simulink model "IEEE_1547_Testing_PHIL"  (R2023b)
settings: Solver=ode4  StartTime=0.0  StopTime=inf  FixedStep=Ts  RelTol=1e-3
PostLoadFcn:
  | init;
InitFcn:
  | init;
undefined symbols (not defined in the file): another_event_name, CURRENT_INPUT_OFFSET_PHA, CURRENT_INPUT_OFFSET_PHB, CURRENT_INPUT_OFFSET_PHC, CURRENT_INPUT_SCALE_PHA, CURRENT_INPUT_SCALE_PHB, CURRENT_INPUT_SCALE_PHC, DiscIntNeverNeededParam, ENABLE_PHA, ENABLE_PHB, ENABLE_PHC, EX, FNOM, FREQUENCY, FREQUENCY_MAX_LIMIT, FREQUENCY_MIN_LIMIT, FRT_CONDITION, FRT_END_TIMING, FRT_START_TIMING, FRT_VALUES, gcbh, magnitude, MODE, my_event_name, Newton, PCRT_CONDITION, PCRT_END_TIMING, PCRT_START_TIMING, PCRT_VALUES, PHASE, PHNOM, Pnom, Raphson, RMS_ENABLE, ROCOF_ENABLE, ROCOF_INIT, ROCOF_VALUE, ROCOM_ENABLE, ROCOM_END_TIME, ROCOM_INIT, ROCOM_START_TIME, ROCOM_VALUE, sps_rtmsupport, Srated, TE0741_4, Ts, TwoSSS_AIO_CPWM, VNOM, VOLT_INPUT_OFFSET_PHA, VOLT_INPUT_OFFSET_PHB, VOLT_INPUT_OFFSET_PHC, VOLT_INPUT_SCALE_PHA, VOLT_INPUT_SCALE_PHB, VOLT_INPUT_SCALE_PHC, VOLT_OUTPUT_SCALE_PHA, VOLT_OUTPUT_SCALE_PHB, VOLT_OUTPUT_SCALE_PHC, VOLTAGE, VOLTAGE_MAX_LIMIT, VOLTAGE_MIN_LIMIT ... (+8)
libraries: simulink x14, rtlab x6, simulink_extras x6, spsFourierLib x6, spsMeanLib x6, rtio_opalrt_common x4, eePowerMeasurement x3, spsPLL3phLib x1, spspowerguiLib x1
(part 2 of 2)

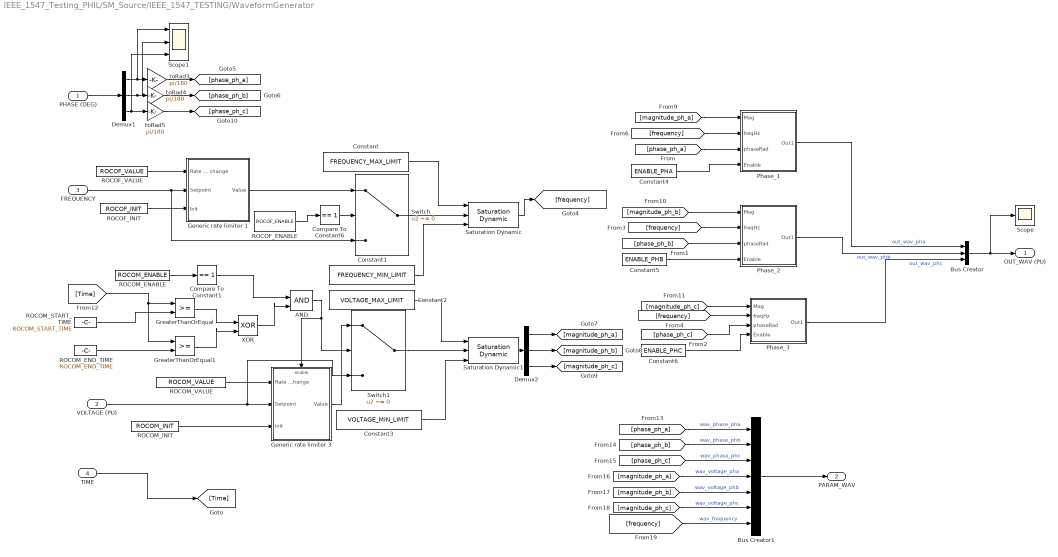
== system IEEE_1547_Testing_PHIL/SM_Source/IEEE_1547_TESTING/WaveformGenerator ==
  PHASE (DEG) : Inport
  VOLTAGE (PU) : Inport  Port=2
  FREQUENCY : Inport  Port=3
  TIME : Inport  Port=4
  AND : Logic  IconShape=distinctive  AllPortsSameDT=off  OutDataTypeStr=boolean
  Bus Creator : BusCreator  Inputs=3
  Bus Creator1 : BusCreator  Inputs=7
  Compare To Constant1 : simulink/Logic and Bit Operations/Compare To Constant  relop===  const=1  OutDataTypeStr=boolean
  Compare To Constant6 : simulink/Logic and Bit Operations/Compare To Constant  relop===  const=1  OutDataTypeStr=boolean
  Constant : Constant  Value=FREQUENCY_MAX_LIMIT
  Constant1 : Constant  Value=FREQUENCY_MIN_LIMIT
  Constant2 : Constant  Value=VOLTAGE_MAX_LIMIT
  Constant3 : Constant  Value=VOLTAGE_MIN_LIMIT
  Constant4 : Constant  Value=ENABLE_PHA
  Constant5 : Constant  Value=ENABLE_PHB
  Constant6 : Constant  Value=ENABLE_PHC
  Demux1 : Demux  Outputs=3
  Demux2 : Demux  Outputs=3
  Generic rate limiter 1 : Subsystem
  Generic rate limiter 3 : Subsystem
  GreaterThanOrEqual : RelationalOperator  OutDataTypeStr=boolean  RndMeth=Simplest  InputSameDT=off
  GreaterThanOrEqual1 : RelationalOperator  OutDataTypeStr=boolean  RndMeth=Simplest  InputSameDT=off
  Phase_1 : Subsystem
  Phase_2 : Subsystem
  Phase_3 : Subsystem
  ROCOF_ENABLE : Constant  Value=ROCOF_ENABLE
  ROCOF_INIT : Constant  Value=ROCOF_INIT
  ROCOF_VALUE : Constant  Value=ROCOF_VALUE
  ROCOM_ENABLE : Constant  Value=ROCOM_ENABLE
  ROCOM_END_TIME : Constant  Value=ROCOM_END_TIME
  ROCOM_INIT : Constant  Value=ROCOM_INIT
  ROCOM_START_TIME : Constant  Value=ROCOM_START_TIME
  ROCOM_VALUE : Constant  Value=ROCOM_VALUE
  Saturation Dynamic : simulink/Discontinuities/Saturation Dynamic  OutMin=[]  OutMax=[]  OutDataTypeStr=Inherit: Same as second input  OutDataType=fixdt(1, 16)  OutScaling=2^-10  DoSatur=off
  Saturation Dynamic1 : simulink/Discontinuities/Saturation Dynamic  OutMin=[]  OutMax=[]  OutDataTypeStr=Inherit: Same as second input  OutDataType=fixdt(1, 16)  OutScaling=2^-10  DoSatur=off
  Scope : Scope
  Scope1 : Scope  NumInputPorts=3
  Switch : Switch  Criteria=u2 ~= 0  SaturateOnIntegerOverflow=off  InputSameDT=off
  Switch1 : Switch  Criteria=u2 ~= 0  SaturateOnIntegerOverflow=off  InputSameDT=off
  XOR : Logic  Operator=XOR  IconShape=distinctive  AllPortsSameDT=off  OutDataTypeStr=boolean
  toRad3 : Gain  Gain=pi/180
  toRad4 : Gain  Gain=pi/180
  toRad5 : Gain  Gain=pi/180
  OUT_WAV (PU) : Outport
  PARAM_WAV : Outport  Port=2
  wires:
  VOLTAGE (PU)/1 -> Switch1/3, Generic rate limiter 3/2("Setpoint ")
  [phase_ph_a] -> Phase_1/3(phaseRad)
  [phase_ph_b] -> Phase_2/3(phaseRad)
  [phase_ph_c] -> Phase_3/3(phaseRad)
  Generic rate limiter 1/1(Value) -> Switch/1
  FREQUENCY/1 -> Switch/3, Generic rate limiter 1/2("Setpoint ")
  ROCOF_VALUE/1 -> Generic rate limiter 1/1(Rate of change)
  ROCOF_INIT/1 -> Generic rate limiter 1/3(Init)
  ROCOF_ENABLE/1 -> Compare To Constant6/1
  Compare To Constant6/1 -> Switch/2
  ROCOM_VALUE/1 -> Generic rate limiter 3/1(Rate of change)
  ROCOM_INIT/1 -> Generic rate limiter 3/3(Init)
  [frequency] -> Phase_1/2(freqHz)
  [frequency] -> Phase_2/2(freqHz)
  Demux2/1 -> [magnitude_ph_a]
  Demux2/2 -> [magnitude_ph_b]
  Demux2/3 -> [magnitude_ph_c]
  [magnitude_ph_a] -> Phase_1/1(Mag)
  [magnitude_ph_b] -> Phase_2/1(Mag)
  [magnitude_ph_c] -> Phase_3/1(Mag)
  [Time] -> GreaterThanOrEqual1/1, GreaterThanOrEqual/1
  ROCOM_START_TIME/1 -> GreaterThanOrEqual/2
  ROCOM_END_TIME/1 -> GreaterThanOrEqual1/2
  GreaterThanOrEqual/1 -> XOR/1
  GreaterThanOrEqual1/1 -> XOR/2
  Switch1/1 -> Saturation Dynamic1/2
  Generic rate limiter 3/1(Value) -> Switch1/1
  AND/1 -> Switch1/2, Generic rate limiter 3/Enable
  XOR/1 -> AND/2
  Compare To Constant1/1 -> AND/1
  ROCOM_ENABLE/1 -> Compare To Constant1/1
  Switch/1 -> Saturation Dynamic/2
  TIME/1 -> [Time]
  Phase_1/1(Out1) -> Bus Creator/1  "out_wav_pha"
  Phase_2/1(Out1) -> Bus Creator/2  "out_wav_phb"
  Phase_3/1(Out1) -> Bus Creator/3  "out_wav_phc"
  Bus Creator/1 -> Scope/1, OUT_WAV (PU)/1
  [phase_ph_a] -> Bus Creator1/1  "wav_phase_pha"
  [phase_ph_b] -> Bus Creator1/2  "wav_phase_phb"
  [phase_ph_c] -> Bus Creator1/3  "wav_phase_phc"
  [magnitude_ph_a] -> Bus Creator1/4  "wav_voltage_pha"
  [magnitude_ph_b] -> Bus Creator1/5  "wav_voltage_phb"
  [magnitude_ph_c] -> Bus Creator1/6  "wav_voltage_phc"
  [frequency] -> Bus Creator1/7  "wav_frequency"
  Bus Creator1/1 -> PARAM_WAV/1
  Saturation Dynamic/1 -> [frequency]
  Saturation Dynamic1/1 -> Demux2/1
  Constant/1 -> Saturation Dynamic/1
  Constant1/1 -> Saturation Dynamic/3
  Constant2/1 -> Saturation Dynamic1/1
  Constant3/1 -> Saturation Dynamic1/3
  Constant4/1 -> Phase_1/4(Enable)
  Constant5/1 -> Phase_2/4(Enable)
  [frequency] -> Phase_3/2(freqHz)
  Constant6/1 -> Phase_3/4(Enable)
  toRad4/1 -> [phase_ph_b]
  toRad3/1 -> [phase_ph_a]
  toRad5/1 -> [phase_ph_c]
  Demux1/2 -> Scope1/2, toRad4/1
  PHASE (DEG)/1 -> Demux1/1
  Demux1/3 -> toRad5/1, Scope1/3
  Demux1/1 -> Scope1/1, toRad3/1

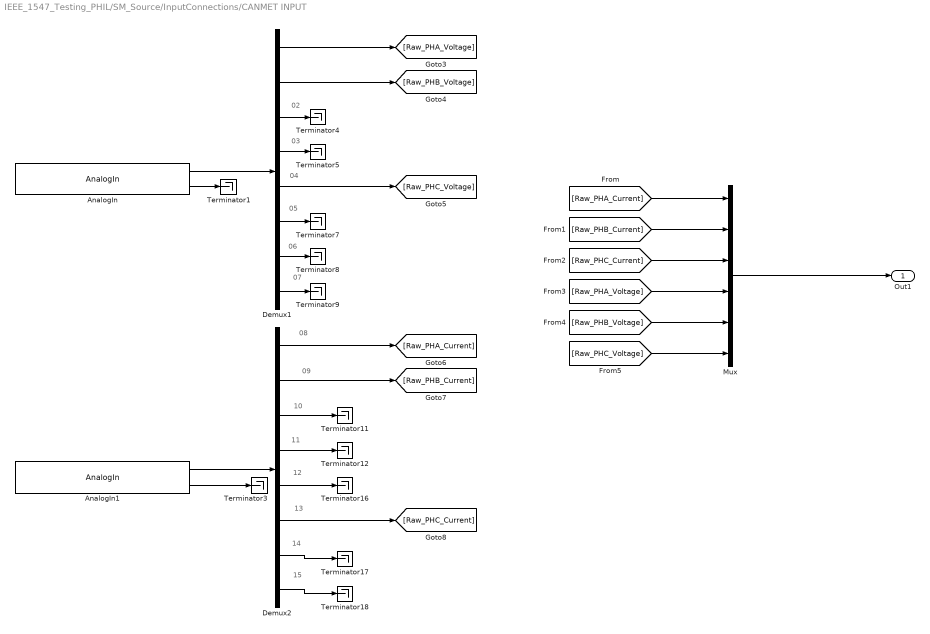
== system IEEE_1547_Testing_PHIL/SM_Source/InputConnections/CANMET INPUT ==
  note: 10
  note: 08
  note: 03
  note: 04
  note: 15
  note: 12
  note: 09
  note: 06
  note: 11
  note: 07
  note: 05
  note: 02
  note: 13
  note: 14
  AnalogIn : rtio_opalrt_common/AnalogIn  CtrlName='OpCtrl'  portNb=7  FcnNos=Slot 6 Module A Subsection 1  size=16  maxcount=8  count=8  numchan=8  sampleTime=0
      settings: AttributesFormatString=%<CtrlName>  SourceProductName=RT-LAB I/O
  AnalogIn1 : rtio_opalrt_common/AnalogIn  CtrlName='OpCtrl'  portNb=8  FcnNos=Slot 6 Module A Subsection 2  size=16  maxcount=8  count=8  numchan=8  sampleTime=0
      settings: AttributesFormatString=%<CtrlName>  SourceProductName=RT-LAB I/O
  Demux1 : Demux  Outputs=8
  Demux2 : Demux  Outputs=8
  Mux : Mux  Inputs=6
  Terminator{1,3..5,7..9,11..12,16..18} (12 alike) : Terminator
  Out1 : Outport  VectorParamsAs1DForOutWhenUnconnected=off
  wires:
  AnalogIn/2 -> Terminator1/1
  AnalogIn1/2 -> Terminator3/1
  AnalogIn/1 -> Demux1/1
  Demux1/4 -> Terminator5/1
  Demux1/7 -> Terminator8/1
  Demux1/6 -> Terminator7/1
  Demux1/8 -> Terminator9/1
  Demux1/3 -> Terminator4/1
  AnalogIn1/1 -> Demux2/1
  Demux2/4 -> Terminator12/1
  Demux2/3 -> Terminator11/1
  Demux2/7 -> Terminator17/1
  Demux2/8 -> Terminator18/1
  Demux2/1 -> [Raw_PHA_Current]
  Demux2/2 -> [Raw_PHB_Current]
  Demux1/5 -> [Raw_PHC_Voltage]
  Demux1/1 -> [Raw_PHA_Voltage]
  Demux1/2 -> [Raw_PHB_Voltage]
  [Raw_PHC_Current] -> Mux/3
  [Raw_PHB_Current] -> Mux/2
  [Raw_PHA_Current] -> Mux/1
  [Raw_PHA_Voltage] -> Mux/4
  [Raw_PHB_Voltage] -> Mux/5
  [Raw_PHC_Voltage] -> Mux/6
  Mux/1 -> Out1/1
  Demux2/5 -> Terminator16/1
  Demux2/6 -> [Raw_PHC_Current]

== system IEEE_1547_Testing_PHIL/SM_Source/IEEE_1547_TESTING/DataAcquisitionSystem/Subsystem ==
  In1 : Inport
  Enable : EnablePort
  FILE_LIMIT : Gain
  FILE_STATUS : Gain
  OpWriteFile : rtlab/DataLogging/OpWriteFile  Static_File=on  varname=Data  Filename=Data.mat  rtpath='./'  nrtpath='.\'  Acq_Group=27  file_size=2.6112e07  write_offline=off  Sim_Mode=off  Nb_Samples=1000  Buffer_size=136000
      settings: SourceProductName=RT-LAB  Decimation=25
  Terminator : Terminator
  Terminator1 : Terminator
  wires:
  OpWriteFile/1 -> FILE_LIMIT/1
  FILE_LIMIT/1 -> Terminator/1
  OpWriteFile/2 -> FILE_STATUS/1
  FILE_STATUS/1 -> Terminator1/1
  In1/1 -> OpWriteFile/1

== system IEEE_1547_Testing_PHIL/SM_Source/IEEE_1547_TESTING/DataAcquisitionSystem/Subsystem1 ==
  In1 : Inport
  Enable : EnablePort
  FILE_LIMIT : Gain
  FILE_STATUS : Gain
  OpWriteFile : rtlab/DataLogging/OpWriteFile  Static_File=on  varname=Data  Filename=WAV.mat  rtpath='./'  nrtpath='.\'  Acq_Group=28  file_size=3e+8  write_offline=off  Sim_Mode=off  Nb_Samples=1000  Buffer_size=200000
      settings: SourceProductName=RT-LAB  Decimation=4
  Terminator : Terminator
  Terminator1 : Terminator
  wires:
  In1/1 -> OpWriteFile/1
  FILE_STATUS/1 -> Terminator1/1
  OpWriteFile/2 -> FILE_STATUS/1
  FILE_LIMIT/1 -> Terminator/1
  OpWriteFile/1 -> FILE_LIMIT/1

== system IEEE_1547_Testing_PHIL/SM_Source/IEEE_1547_TESTING/SignalConditionning/RMS1 ==
  In : Inport  SampleTime=Ts
  Constant : Constant  Value=TrueRMS
  Data Type Conversion : DataTypeConversion  OutDataTypeStr=boolean  SaturateOnIntegerOverflow=off  RndMeth=Floor
  Logical Operator : Logic  Operator=NOT  AllPortsSameDT=off  OutDataTypeStr=boolean
  "RMS " : Subsystem
  Switch : Switch  Criteria=u2 ~= 0  Threshold=0.5  SaturateOnIntegerOverflow=off  InputSameDT=off
  "TrueRMS " : Subsystem
  RMS : Outport  PortDimensions=1  SampleTime=Ts  VectorParamsAs1DForOutWhenUnconnected=off
  wires:
  In/1 -> "TrueRMS "/1(In), "RMS "/1(In)
  Switch/1 -> RMS/1
  "TrueRMS "/1(RMS) -> Switch/1
  "RMS "/1(RMS) -> Switch/3
  Constant/1 -> Data Type Conversion/1
  Data Type Conversion/1 -> Logical Operator/1, "TrueRMS "/Enable, Switch/2
  Logical Operator/1 -> "RMS "/Enable

== system IEEE_1547_Testing_PHIL/SM_Source/IEEE_1547_TESTING/SignalConditionning/RMS2 ==
  In : Inport  SampleTime=Ts
  Constant : Constant  Value=TrueRMS
  Data Type Conversion : DataTypeConversion  OutDataTypeStr=boolean  SaturateOnIntegerOverflow=off  RndMeth=Floor
  Logical Operator : Logic  Operator=NOT  AllPortsSameDT=off  OutDataTypeStr=boolean
  "RMS " : Subsystem
  Switch : Switch  Criteria=u2 ~= 0  Threshold=0.5  SaturateOnIntegerOverflow=off  InputSameDT=off
  "TrueRMS " : Subsystem
  RMS : Outport  PortDimensions=1  SampleTime=Ts  VectorParamsAs1DForOutWhenUnconnected=off
  wires:
  In/1 -> "TrueRMS "/1(In), "RMS "/1(In)
  Switch/1 -> RMS/1
  "TrueRMS "/1(RMS) -> Switch/1
  "RMS "/1(RMS) -> Switch/3
  Constant/1 -> Data Type Conversion/1
  Data Type Conversion/1 -> Logical Operator/1, "TrueRMS "/Enable, Switch/2
  Logical Operator/1 -> "RMS "/Enable

== system IEEE_1547_Testing_PHIL/SM_Source/IEEE_1547_TESTING/SignalConditionning/RMS3 ==
  In : Inport  SampleTime=Ts
  Constant : Constant  Value=TrueRMS
  Data Type Conversion : DataTypeConversion  OutDataTypeStr=boolean  SaturateOnIntegerOverflow=off  RndMeth=Floor
  Logical Operator : Logic  Operator=NOT  AllPortsSameDT=off  OutDataTypeStr=boolean
  "RMS " : Subsystem
  Switch : Switch  Criteria=u2 ~= 0  Threshold=0.5  SaturateOnIntegerOverflow=off  InputSameDT=off
  "TrueRMS " : Subsystem
  RMS : Outport  PortDimensions=1  SampleTime=Ts  VectorParamsAs1DForOutWhenUnconnected=off
  wires:
  In/1 -> "TrueRMS "/1(In), "RMS "/1(In)
  Switch/1 -> RMS/1
  "TrueRMS "/1(RMS) -> Switch/1
  "RMS "/1(RMS) -> Switch/3
  Constant/1 -> Data Type Conversion/1
  Data Type Conversion/1 -> Logical Operator/1, "TrueRMS "/Enable, Switch/2
  Logical Operator/1 -> "RMS "/Enable

== system IEEE_1547_Testing_PHIL/SM_Source/IEEE_1547_TESTING/SignalConditionning/RMS4 ==
  In : Inport  SampleTime=Ts
  Constant : Constant  Value=TrueRMS
  Data Type Conversion : DataTypeConversion  OutDataTypeStr=boolean  SaturateOnIntegerOverflow=off  RndMeth=Floor
  Logical Operator : Logic  Operator=NOT  AllPortsSameDT=off  OutDataTypeStr=boolean
  "RMS " : Subsystem
  Switch : Switch  Criteria=u2 ~= 0  Threshold=0.5  SaturateOnIntegerOverflow=off  InputSameDT=off
  "TrueRMS " : Subsystem
  RMS : Outport  PortDimensions=1  SampleTime=Ts  VectorParamsAs1DForOutWhenUnconnected=off
  wires:
  In/1 -> "TrueRMS "/1(In), "RMS "/1(In)
  Switch/1 -> RMS/1
  "TrueRMS "/1(RMS) -> Switch/1
  "RMS "/1(RMS) -> Switch/3
  Constant/1 -> Data Type Conversion/1
  Data Type Conversion/1 -> Logical Operator/1, "TrueRMS "/Enable, Switch/2
  Logical Operator/1 -> "RMS "/Enable

== system IEEE_1547_Testing_PHIL/SM_Source/IEEE_1547_TESTING/SignalConditionning/RMS6 ==
  In : Inport  SampleTime=Ts
  Constant : Constant  Value=TrueRMS
  Data Type Conversion : DataTypeConversion  OutDataTypeStr=boolean  SaturateOnIntegerOverflow=off  RndMeth=Floor
  Logical Operator : Logic  Operator=NOT  AllPortsSameDT=off  OutDataTypeStr=boolean
  "RMS " : Subsystem
  Switch : Switch  Criteria=u2 ~= 0  Threshold=0.5  SaturateOnIntegerOverflow=off  InputSameDT=off
  "TrueRMS " : Subsystem
  RMS : Outport  PortDimensions=1  SampleTime=Ts  VectorParamsAs1DForOutWhenUnconnected=off
  wires:
  In/1 -> "TrueRMS "/1(In), "RMS "/1(In)
  Switch/1 -> RMS/1
  "TrueRMS "/1(RMS) -> Switch/1
  "RMS "/1(RMS) -> Switch/3
  Constant/1 -> Data Type Conversion/1
  Data Type Conversion/1 -> Logical Operator/1, "TrueRMS "/Enable, Switch/2
  Logical Operator/1 -> "RMS "/Enable

== system IEEE_1547_Testing_PHIL/SM_Source/IEEE_1547_TESTING/SignalConditionning/RMS7 ==
  In : Inport  SampleTime=Ts
  Constant : Constant  Value=TrueRMS
  Data Type Conversion : DataTypeConversion  OutDataTypeStr=boolean  SaturateOnIntegerOverflow=off  RndMeth=Floor
  Logical Operator : Logic  Operator=NOT  AllPortsSameDT=off  OutDataTypeStr=boolean
  "RMS " : Subsystem
  Switch : Switch  Criteria=u2 ~= 0  Threshold=0.5  SaturateOnIntegerOverflow=off  InputSameDT=off
  "TrueRMS " : Subsystem
  RMS : Outport  PortDimensions=1  SampleTime=Ts  VectorParamsAs1DForOutWhenUnconnected=off
  wires:
  In/1 -> "TrueRMS "/1(In), "RMS "/1(In)
  Switch/1 -> RMS/1
  "TrueRMS "/1(RMS) -> Switch/1
  "RMS "/1(RMS) -> Switch/3
  Constant/1 -> Data Type Conversion/1
  Data Type Conversion/1 -> Logical Operator/1, "TrueRMS "/Enable, Switch/2
  Logical Operator/1 -> "RMS "/Enable

== system IEEE_1547_Testing_PHIL/SM_Source/IEEE_1547_TESTING/SignalConditionning/Subsystem ==
  P : Inport
  Q : Inport  Port=2
  Divide : Product  Inputs=*/
  Math Function6 : Math  Operator=hypot  SignedPower=on
  Saturation : Saturate  UpperLimit=1.1  LowerLimit=0
  PF : Outport  VectorParamsAs1DForOutWhenUnconnected=off
  wires:
  Divide/1 -> Saturation/1
  P/1 -> Divide/1, Math Function6/1
  Q/1 -> Math Function6/2
  Math Function6/1 -> Divide/2
  Saturation/1 -> PF/1

== system IEEE_1547_Testing_PHIL/SM_Source/IEEE_1547_TESTING/SignalConditionning/Subsystem1 ==
  P : Inport
  Q : Inport  Port=2
  Divide : Product  Inputs=*/
  Math Function6 : Math  Operator=hypot  SignedPower=on
  Saturation : Saturate  UpperLimit=1.1  LowerLimit=0
  PF : Outport  VectorParamsAs1DForOutWhenUnconnected=off
  wires:
  Saturation/1 -> PF/1
  Math Function6/1 -> Divide/2
  Q/1 -> Math Function6/2
  P/1 -> Math Function6/1, Divide/1
  Divide/1 -> Saturation/1

== system IEEE_1547_Testing_PHIL/SM_Source/IEEE_1547_TESTING/SignalConditionning/Subsystem2 ==
  P : Inport
  Q : Inport  Port=2
  Divide : Product  Inputs=*/
  Math Function6 : Math  Operator=hypot  SignedPower=on
  Saturation : Saturate  UpperLimit=1.1  LowerLimit=0
  PF : Outport  VectorParamsAs1DForOutWhenUnconnected=off
  wires:
  Divide/1 -> Saturation/1
  P/1 -> Divide/1, Math Function6/1
  Q/1 -> Math Function6/2
  Math Function6/1 -> Divide/2
  Saturation/1 -> PF/1

== system IEEE_1547_Testing_PHIL/SM_Source/IEEE_1547_TESTING/WaveformGenerator/Generic rate limiter 1 ==
  Rate of change : Inport
  "Setpoint " : Inport  Port=2
  Init : Inport  Port=3
  Add1 : Sum  Inputs=+-
  Add2 : Sum
  Gain : Gain  Gain=-1
  Rate Limiter Dynamic : simulink/Discontinuities/Rate Limiter Dynamic
  Value : Outport  VectorParamsAs1DForOutWhenUnconnected=off
  wires:
  Rate Limiter Dynamic/1 -> Add2/1  "Freq"
  Add2/1 -> Value/1  "Freq"
  Gain/1 -> Rate Limiter Dynamic/3
  Add1/1 -> Rate Limiter Dynamic/2
  "Setpoint "/1 -> Add1/1
  Rate of change/1 -> Gain/1, Rate Limiter Dynamic/1
  Init/1 -> Add1/2, Add2/2

== system IEEE_1547_Testing_PHIL/SM_Source/IEEE_1547_TESTING/WaveformGenerator/Generic rate limiter 3 ==
  Rate of change : Inport
  "Setpoint " : Inport  Port=2
  Init : Inport  Port=3
  Enable : EnablePort
  Add1 : Sum  Inputs=+-
  Add2 : Sum
  Gain : Gain  Gain=-1
  Rate Limiter Dynamic : simulink/Discontinuities/Rate Limiter Dynamic
  Value : Outport  VectorParamsAs1DForOutWhenUnconnected=off
  wires:
  Init/1 -> Add2/2, Add1/2
  Rate of change/1 -> Rate Limiter Dynamic/1, Gain/1
  "Setpoint "/1 -> Add1/1
  Add1/1 -> Rate Limiter Dynamic/2
  Gain/1 -> Rate Limiter Dynamic/3
  Add2/1 -> Value/1
  Rate Limiter Dynamic/1 -> Add2/1

== system IEEE_1547_Testing_PHIL/SM_Source/IEEE_1547_TESTING/WaveformGenerator/Phase_1 ==
  Mag : Inport
  freqHz : Inport  Port=2
  phaseRad : Inport  Port=3
  Enable : Inport  Port=4
  2pi : Gain  Gain=2*pi
  Add : Sum
  Constant : Constant  Value=0
  Discrete-Time Integrator : DiscreteIntegrator  SampleTime=Ts  ICPrevOutput=DiscIntNeverNeededParam  ICPrevScaledInput=DiscIntNeverNeededParam
  Product1 : Product
  Scope : Scope
  Switch : Switch  Criteria=u2 > Threshold  SaturateOnIntegerOverflow=off  InputSameDT=off
  Trigonometric Function : Trigonometry  Operator=cos  OutputSignalType=real
  Out1 : Outport  VectorParamsAs1DForOutWhenUnconnected=off
  wires:
  Mag/1 -> Product1/1
  Trigonometric Function/1 -> Scope/1, Product1/2
  freqHz/1 -> 2pi/1  "f"
  phaseRad/1 -> Add/2  "phi"
  Product1/1 -> Switch/1
  2pi/1 -> Discrete-Time Integrator/1  "w"
  Discrete-Time Integrator/1 -> Add/1  "wt"
  Add/1 -> Trigonometric Function/1  "wt+phi"
  Enable/1 -> Switch/2
  Switch/1 -> Out1/1
  Constant/1 -> Switch/3

== system IEEE_1547_Testing_PHIL/SM_Source/IEEE_1547_TESTING/WaveformGenerator/Phase_2 ==
  Mag : Inport
  freqHz : Inport  Port=2
  phaseRad : Inport  Port=3
  Enable : Inport  Port=4
  2pi : Gain  Gain=2*pi
  Add : Sum
  Constant : Constant  Value=0
  Discrete-Time Integrator : DiscreteIntegrator  SampleTime=Ts  ICPrevOutput=DiscIntNeverNeededParam  ICPrevScaledInput=DiscIntNeverNeededParam
  Product1 : Product
  Scope : Scope
  Switch : Switch  Criteria=u2 > Threshold  SaturateOnIntegerOverflow=off  InputSameDT=off
  Trigonometric Function : Trigonometry  Operator=cos  OutputSignalType=real
  Out1 : Outport  VectorParamsAs1DForOutWhenUnconnected=off
  wires:
  Constant/1 -> Switch/3
  Switch/1 -> Out1/1
  Enable/1 -> Switch/2
  Add/1 -> Trigonometric Function/1  "wt+phi"
  Discrete-Time Integrator/1 -> Add/1  "wt"
  2pi/1 -> Discrete-Time Integrator/1  "w"
  Product1/1 -> Switch/1
  phaseRad/1 -> Add/2  "phi"
  freqHz/1 -> 2pi/1  "f"
  Trigonometric Function/1 -> Product1/2, Scope/1
  Mag/1 -> Product1/1

== system IEEE_1547_Testing_PHIL/SM_Source/IEEE_1547_TESTING/WaveformGenerator/Phase_3 ==
  Mag : Inport
  freqHz : Inport  Port=2
  phaseRad : Inport  Port=3
  Enable : Inport  Port=4
  2pi : Gain  Gain=2*pi
  Add : Sum
  Constant : Constant  Value=0
  Discrete-Time Integrator : DiscreteIntegrator  SampleTime=Ts  ICPrevOutput=DiscIntNeverNeededParam  ICPrevScaledInput=DiscIntNeverNeededParam
  Product1 : Product
  Scope : Scope
  Switch : Switch  Criteria=u2 > Threshold  SaturateOnIntegerOverflow=off  InputSameDT=off
  Trigonometric Function : Trigonometry  Operator=cos  OutputSignalType=real
  Out1 : Outport  VectorParamsAs1DForOutWhenUnconnected=off
  wires:
  Mag/1 -> Product1/1
  Trigonometric Function/1 -> Scope/1, Product1/2
  freqHz/1 -> 2pi/1  "f"
  phaseRad/1 -> Add/2  "phi"
  Product1/1 -> Switch/1
  2pi/1 -> Discrete-Time Integrator/1  "w"
  Discrete-Time Integrator/1 -> Add/1  "wt"
  Add/1 -> Trigonometric Function/1  "wt+phi"
  Enable/1 -> Switch/2
  Switch/1 -> Out1/1
  Constant/1 -> Switch/3

== system IEEE_1547_Testing_PHIL/SM_Source/IEEE_1547_TESTING/SignalConditionning/RMS1/RMS  ==
  In : Inport
  Enable : EnablePort
  Fourier1 : spsFourierLib/Fourier  Freq=sps.Freq  n=1  InInit=sps.Par_Init_RMS  Ts=Ts
  Gain : Gain  Gain=1/sqrt(2)
  Terminator : Terminator
  RMS : Outport  VectorParamsAs1DForOutWhenUnconnected=off
  wires:
  Fourier1/1 -> Gain/1
  Fourier1/2 -> Terminator/1
  In/1 -> Fourier1/1
  Gain/1 -> RMS/1

== system IEEE_1547_Testing_PHIL/SM_Source/IEEE_1547_TESTING/SignalConditionning/RMS1/TrueRMS  ==
  In : Inport
  Enable : EnablePort
  Mean value : spsMeanLib/Mean  Freq=sps.Freq  Vinit=sps.Par_Init_TrueRMS  Ts=Ts
  Product : Product  InputSameDT=on  SaturateOnIntegerOverflow=on  OutDataTypeStr=Inherit: Same as first input
  Saturation to avoid negative sqrt : Saturate  UpperLimit=Inf  LowerLimit=0
  Sqrt : Sqrt  AlgorithmType=Newton-Raphson
  RMS : Outport  VectorParamsAs1DForOutWhenUnconnected=off
  wires:
  Saturation to avoid negative sqrt/1 -> Sqrt/1
  Mean value/1 -> Saturation to avoid negative sqrt/1
  Product/1 -> Mean value/1
  In/1 -> Product/2, Product/1
  Sqrt/1 -> RMS/1

== system IEEE_1547_Testing_PHIL/SM_Source/IEEE_1547_TESTING/SignalConditionning/RMS2/RMS  ==
  In : Inport
  Enable : EnablePort
  Fourier1 : spsFourierLib/Fourier  Freq=sps.Freq  n=1  InInit=sps.Par_Init_RMS  Ts=Ts
  Gain : Gain  Gain=1/sqrt(2)
  Terminator : Terminator
  RMS : Outport  VectorParamsAs1DForOutWhenUnconnected=off
  wires:
  Fourier1/1 -> Gain/1
  Fourier1/2 -> Terminator/1
  In/1 -> Fourier1/1
  Gain/1 -> RMS/1

== system IEEE_1547_Testing_PHIL/SM_Source/IEEE_1547_TESTING/SignalConditionning/RMS2/TrueRMS  ==
  In : Inport
  Enable : EnablePort
  Mean value : spsMeanLib/Mean  Freq=sps.Freq  Vinit=sps.Par_Init_TrueRMS  Ts=Ts
  Product : Product  InputSameDT=on  SaturateOnIntegerOverflow=on  OutDataTypeStr=Inherit: Same as first input
  Saturation to avoid negative sqrt : Saturate  UpperLimit=Inf  LowerLimit=0
  Sqrt : Sqrt  AlgorithmType=Newton-Raphson
  RMS : Outport  VectorParamsAs1DForOutWhenUnconnected=off
  wires:
  Saturation to avoid negative sqrt/1 -> Sqrt/1
  Mean value/1 -> Saturation to avoid negative sqrt/1
  Product/1 -> Mean value/1
  In/1 -> Product/2, Product/1
  Sqrt/1 -> RMS/1

== system IEEE_1547_Testing_PHIL/SM_Source/IEEE_1547_TESTING/SignalConditionning/RMS3/RMS  ==
  In : Inport
  Enable : EnablePort
  Fourier1 : spsFourierLib/Fourier  Freq=sps.Freq  n=1  InInit=sps.Par_Init_RMS  Ts=Ts
  Gain : Gain  Gain=1/sqrt(2)
  Terminator : Terminator
  RMS : Outport  VectorParamsAs1DForOutWhenUnconnected=off
  wires:
  Fourier1/1 -> Gain/1
  Fourier1/2 -> Terminator/1
  In/1 -> Fourier1/1
  Gain/1 -> RMS/1

== system IEEE_1547_Testing_PHIL/SM_Source/IEEE_1547_TESTING/SignalConditionning/RMS3/TrueRMS  ==
  In : Inport
  Enable : EnablePort
  Mean value : spsMeanLib/Mean  Freq=sps.Freq  Vinit=sps.Par_Init_TrueRMS  Ts=Ts
  Product : Product  InputSameDT=on  SaturateOnIntegerOverflow=on  OutDataTypeStr=Inherit: Same as first input
  Saturation to avoid negative sqrt : Saturate  UpperLimit=Inf  LowerLimit=0
  Sqrt : Sqrt  AlgorithmType=Newton-Raphson
  RMS : Outport  VectorParamsAs1DForOutWhenUnconnected=off
  wires:
  Saturation to avoid negative sqrt/1 -> Sqrt/1
  Mean value/1 -> Saturation to avoid negative sqrt/1
  Product/1 -> Mean value/1
  In/1 -> Product/2, Product/1
  Sqrt/1 -> RMS/1

== system IEEE_1547_Testing_PHIL/SM_Source/IEEE_1547_TESTING/SignalConditionning/RMS4/RMS  ==
  In : Inport
  Enable : EnablePort
  Fourier1 : spsFourierLib/Fourier  Freq=sps.Freq  n=1  InInit=sps.Par_Init_RMS  Ts=Ts
  Gain : Gain  Gain=1/sqrt(2)
  Terminator : Terminator
  RMS : Outport  VectorParamsAs1DForOutWhenUnconnected=off
  wires:
  Fourier1/1 -> Gain/1
  Fourier1/2 -> Terminator/1
  In/1 -> Fourier1/1
  Gain/1 -> RMS/1

== system IEEE_1547_Testing_PHIL/SM_Source/IEEE_1547_TESTING/SignalConditionning/RMS4/TrueRMS  ==
  In : Inport
  Enable : EnablePort
  Mean value : spsMeanLib/Mean  Freq=sps.Freq  Vinit=sps.Par_Init_TrueRMS  Ts=Ts
  Product : Product  InputSameDT=on  SaturateOnIntegerOverflow=on  OutDataTypeStr=Inherit: Same as first input
  Saturation to avoid negative sqrt : Saturate  UpperLimit=Inf  LowerLimit=0
  Sqrt : Sqrt  AlgorithmType=Newton-Raphson
  RMS : Outport  VectorParamsAs1DForOutWhenUnconnected=off
  wires:
  Saturation to avoid negative sqrt/1 -> Sqrt/1
  Mean value/1 -> Saturation to avoid negative sqrt/1
  Product/1 -> Mean value/1
  In/1 -> Product/2, Product/1
  Sqrt/1 -> RMS/1

== system IEEE_1547_Testing_PHIL/SM_Source/IEEE_1547_TESTING/SignalConditionning/RMS6/RMS  ==
  In : Inport
  Enable : EnablePort
  Fourier1 : spsFourierLib/Fourier  Freq=sps.Freq  n=1  InInit=sps.Par_Init_RMS  Ts=Ts
  Gain : Gain  Gain=1/sqrt(2)
  Terminator : Terminator
  RMS : Outport  VectorParamsAs1DForOutWhenUnconnected=off
  wires:
  Fourier1/1 -> Gain/1
  Fourier1/2 -> Terminator/1
  In/1 -> Fourier1/1
  Gain/1 -> RMS/1

== system IEEE_1547_Testing_PHIL/SM_Source/IEEE_1547_TESTING/SignalConditionning/RMS6/TrueRMS  ==
  In : Inport
  Enable : EnablePort
  Mean value : spsMeanLib/Mean  Freq=sps.Freq  Vinit=sps.Par_Init_TrueRMS  Ts=Ts
  Product : Product  InputSameDT=on  SaturateOnIntegerOverflow=on  OutDataTypeStr=Inherit: Same as first input
  Saturation to avoid negative sqrt : Saturate  UpperLimit=Inf  LowerLimit=0
  Sqrt : Sqrt  AlgorithmType=Newton-Raphson
  RMS : Outport  VectorParamsAs1DForOutWhenUnconnected=off
  wires:
  Saturation to avoid negative sqrt/1 -> Sqrt/1
  Mean value/1 -> Saturation to avoid negative sqrt/1
  Product/1 -> Mean value/1
  In/1 -> Product/2, Product/1
  Sqrt/1 -> RMS/1

== system IEEE_1547_Testing_PHIL/SM_Source/IEEE_1547_TESTING/SignalConditionning/RMS7/RMS  ==
  In : Inport
  Enable : EnablePort
  Fourier1 : spsFourierLib/Fourier  Freq=sps.Freq  n=1  InInit=sps.Par_Init_RMS  Ts=Ts
  Gain : Gain  Gain=1/sqrt(2)
  Terminator : Terminator
  RMS : Outport  VectorParamsAs1DForOutWhenUnconnected=off
  wires:
  Fourier1/1 -> Gain/1
  Fourier1/2 -> Terminator/1
  In/1 -> Fourier1/1
  Gain/1 -> RMS/1

== system IEEE_1547_Testing_PHIL/SM_Source/IEEE_1547_TESTING/SignalConditionning/RMS7/TrueRMS  ==
  In : Inport
  Enable : EnablePort
  Mean value : spsMeanLib/Mean  Freq=sps.Freq  Vinit=sps.Par_Init_TrueRMS  Ts=Ts
  Product : Product  InputSameDT=on  SaturateOnIntegerOverflow=on  OutDataTypeStr=Inherit: Same as first input
  Saturation to avoid negative sqrt : Saturate  UpperLimit=Inf  LowerLimit=0
  Sqrt : Sqrt  AlgorithmType=Newton-Raphson
  RMS : Outport  VectorParamsAs1DForOutWhenUnconnected=off
  wires:
  Saturation to avoid negative sqrt/1 -> Sqrt/1
  Mean value/1 -> Saturation to avoid negative sqrt/1
  Product/1 -> Mean value/1
  In/1 -> Product/2, Product/1
  Sqrt/1 -> RMS/1

== matlab function IEEE_1547_Testing_PHIL/SM_Source/IEEE_1547_TESTING/FRT/MATLAB Function1 ==
  settings: updateMethod=DISCRETE
  data: TIME input; COMMAND output; CONDITIONS input; START_TIMING input; END_TIMING input; VALUES input; TRIGGER output; TEST_CONDITION output; COMPLETED output; NOMINAL input
function [COMMAND, TRIGGER, TEST_CONDITION, COMPLETED] = disturbances_logic(TIME,CONDITIONS,START_TIMING,END_TIMING,VALUES, NOMINAL)

% all actions are condition actions and 
% outputs are function of state and input 
persistent current_value;
persistent current_state;
persistent current_trigger;
persistent index;
persistent current_test_condition;

% define states
START = 0;
CHECK_TIMING = 1;
NEXT_INDEX = 2;
LAST_INDEX = 3;
COMPLETED_SEQUENCE = 4;
% Define useful variables

% Make sure variables are initialize
if isempty(current_value)
    current_value = NOMINAL; 
end
if isempty(current_state)
    current_state = START; 
end
if isempty(current_trigger)
    current_trigger = 0;   
end
if isempty(index)
    index = 1;   
end
if isempty(current_test_condition)
    current_test_condition = 0;   
end
% Simple state machine to handle iteration base on time
switch (current_state) 
    case START,
        % value of output 'command' depends both on state and inputs
        if (TIME > START_TIMING(index))
            current_state = CHECK_TIMING;
        else
            current_state = START;
            % Start at nominal
            current_value = NOMINAL; 

        end
    case CHECK_TIMING,
        % value of output 'command' depends both on state and inputs
        if (TIME>END_TIMING(index))
            current_state = NEXT_INDEX;
        else
            current_state = CHECK_TIMING;
            current_value = VALUES(index);
            current_test_condition = CONDITIONS(index)
            current_trigger = 1;

        end
    case NEXT_INDEX,
        % value of output 'command' depends both on state and inputs
        index = index + 1 
        if(CONDITIONS(index + 1) == 0)
            current_state = LAST_INDEX;
        else
            current_state = CHECK_TIMING;
        end
    case LAST_INDEX,
        if (TIME>END_TIMING(index))
            current_state = COMPLETED_SEQUENCE;
        else
            current_state = LAST_INDEX;
            current_value = VALUES(index);
            current_test_condition = CONDITIONS(index)

        end
    case COMPLETED_SEQUENCE,
        % Going back to nominal, in case other sequences needed
        current_state = COMPLETED_SEQUENCE;
        current_trigger = 0;
        current_value = NOMINAL; 
        current_test_condition = 0

end
TEST_CONDITION = current_test_condition;
COMMAND = current_value;
TRIGGER = current_trigger;

if (current_state == COMPLETED_SEQUENCE)
    COMPLETED = 1;
else
    COMPLETED = 0;
end

== matlab function IEEE_1547_Testing_PHIL/SM_Source/IEEE_1547_TESTING/PCRT/MATLAB Function1 ==
  settings: updateMethod=DISCRETE
  data: TIME input; COMMAND output; CONDITIONS input; START_TIMING input; END_TIMING input; VALUES input; TRIGGER output; TEST_CONDITION output; COMPLETED output; NOMINAL input
function [COMMAND, TRIGGER, TEST_CONDITION, COMPLETED] = disturbances_logic(TIME,CONDITIONS,START_TIMING,END_TIMING,VALUES, NOMINAL)

% all actions are condition actions and 
% outputs are function of state and input 
persistent current_value;
persistent current_state;
persistent current_trigger;
persistent index;
persistent current_test_condition;

% define states
START = 0;
CHECK_TIMING = 1;
NEXT_INDEX = 2;
LAST_INDEX = 3;
COMPLETED_SEQUENCE = 4;
% Define useful variables

% Make sure variables are initialize
if isempty(current_value)
    current_value = NOMINAL; 
end
if isempty(current_state)
    current_state = START; 
end
if isempty(current_trigger)
    current_trigger = 0;   
end
if isempty(index)
    index = 1;   
end
if isempty(current_test_condition)
    current_test_condition = 0;   
end
% Simple state machine to handle iteration base on time
switch (current_state) 
    case START,
        % value of output 'command' depends both on state and inputs
        if (TIME > START_TIMING(index))
            current_state = CHECK_TIMING;
        else
            current_state = START;
            % Start at nominal
            current_value = NOMINAL; 

        end
    case CHECK_TIMING,
        % value of output 'command' depends both on state and inputs
        if (TIME>END_TIMING(index))
            current_state = NEXT_INDEX;
        else
            current_state = CHECK_TIMING;
            current_test_condition = CONDITIONS(index)
            switch (current_test_condition)
                case 1,
                    current_value = NOMINAL;
                case 2,
                    current_value = NOMINAL + [VALUES(index), 0, 0]';
                case 3,
                    current_value = NOMINAL + [0, VALUES(index), 0]';
                case 4,
                    current_value = NOMINAL + [0, 0, VALUES(index)]';
                case 5,
                    current_value = NOMINAL + VALUES(index);
                case 6,
                    current_value = NOMINAL - VALUES(index);
            end
            
            current_trigger = 1;

        end
    case NEXT_INDEX,
        % value of output 'command' depends both on state and inputs
        index = index + 1 
        if(CONDITIONS(index + 1) == 0)
            current_state = LAST_INDEX;
        else
            current_state = CHECK_TIMING;
        end
    case LAST_INDEX,
        if (TIME>END_TIMING(index))
            current_state = COMPLETED_SEQUENCE;
        else
            current_state = LAST_INDEX;
            current_test_condition = CONDITIONS(index)
            switch (current_test_condition)
                case 1,
                    current_value = NOMINAL;
                case 2,
                    current_value = NOMINAL + [VALUES(index), 0, 0]';
                case 3,
                    current_value = NOMINAL + [0, VALUES(index), 0]';
                case 4,
                    current_value = NOMINAL + [0, 0, VALUES(index)]';
                case 5,
                    current_value = NOMINAL + VALUES(index);
                 case 6,
                    current_value = NOMINAL - VALUES(index);
            end
        end
    case COMPLETED_SEQUENCE,
        % Going back to nominal, in case other sequences needed
        current_state = COMPLETED_SEQUENCE;
        current_trigger = 0;
        current_value = NOMINAL; 
        current_test_condition = 0

end
TEST_CONDITION = current_test_condition;
COMMAND = current_value;
TRIGGER = current_trigger;

if (current_state == COMPLETED_SEQUENCE)
    COMPLETED = 1;
else
    COMPLETED = 0;
end

== matlab function IEEE_1547_Testing_PHIL/SM_Source/IEEE_1547_TESTING/VRT/MATLAB Function1 ==
  settings: updateMethod=DISCRETE
  data: TIME input; COMMAND output; CONDITIONS input; START_TIMING input; END_TIMING input; VALUES input; TRIGGER output; TEST_CONDITION output; COMPLETED output; NOMINAL input
function [COMMAND, TRIGGER, TEST_CONDITION, COMPLETED] = disturbances_logic(TIME,CONDITIONS,START_TIMING,END_TIMING,VALUES, NOMINAL)

% all actions are condition actions and 
% outputs are function of state and input 
persistent current_value;
persistent current_state;
persistent current_trigger;
persistent index;
persistent current_test_condition;

% define states
START = 0;
CHECK_TIMING = 1;
NEXT_INDEX = 2;
LAST_INDEX = 3;
COMPLETED_SEQUENCE = 4;
% Define useful variables

% Make sure variables are initialize
if isempty(current_value)
    current_value = NOMINAL; 
end
if isempty(current_state)
    current_state = START; 
end
if isempty(current_trigger)
    current_trigger = 0;   
end
if isempty(current_test_condition)
    current_test_condition = 0;   
end
if isempty(index)
    index = 1;   
end
% Simple state machine to handle iteration base on time
switch (current_state) 
    case START,
        % value of output 'command' depends both on state and inputs
        if (TIME > START_TIMING(index))
            current_state = CHECK_TIMING;
        else
            current_state = START;
            % Start at nominal
            current_value = NOMINAL; 

        end
    case CHECK_TIMING,
        % value of output 'command' depends both on state and inputs
        if (TIME>END_TIMING(index))
            current_state = NEXT_INDEX;
        else
            current_state = CHECK_TIMING;
            current_value = VALUES(index);
            current_test_condition = CONDITIONS(index)
            current_trigger = 1;

        end
    case NEXT_INDEX,
        % value of output 'command' depends both on state and inputs
        index = index + 1 
        if(CONDITIONS(index + 1) == 0)
            current_state = LAST_INDEX;
        else
            current_state = CHECK_TIMING;
        end
    case LAST_INDEX,
        if (TIME>END_TIMING(index))
            current_state = COMPLETED_SEQUENCE;
        else
            current_state = LAST_INDEX;
            current_value = VALUES(index);
            current_test_condition = CONDITIONS(index)

        end
    case COMPLETED_SEQUENCE,
        % Going back to nominal, in case other sequences needed
        current_state = COMPLETED_SEQUENCE;
        current_trigger = 0;
        current_value = NOMINAL; 
        current_test_condition = 0

end
TEST_CONDITION = current_test_condition;
COMMAND = current_value;
TRIGGER = current_trigger;


if (current_state == COMPLETED_SEQUENCE)
    COMPLETED = 1;
else
    COMPLETED = 0;
end
